simulink model "Assignment_1"  (R2022b)
settings: Solver=FixedStepAuto  StartTime=0.0  StopTime=10.0  FixedStep=1e-3  RelTol=1e-3  EnableMultiTasking=on
settings Model: ExtModeTrigDuration=5  Creator=rebec  LastModifiedBy=rebec
settings OptimizationCC: EnhancedBackFolding=on  PassReuseOutputArgsAs=Individual arguments  ZeroExternalMemoryAtStartup=off  ZeroInternalMemoryAtStartup=off  MaxStackSize=64  OptimizeBlockOrder=speed  DifferentSizesBufferReuse=on  OptimizationCustomize=off  EfficientTunableParamExpr=on
settings DebuggingCC: ParameterTunabilityLossMsg=error
settings HardwareCC: ProdBitPerPointer=32  ProdBitPerSizeT=32  ProdBitPerPtrDiffT=32  ProdLargestAtomicInteger=Long  ProdLargestAtomicFloat=Double  ProdWordSize=32  ProdHWDeviceType=ARM Compatible->ARM Cortex
settings SFSimCC: MATLABDynamicMemAlloc=off
settings RTWCC: Description=Embedded Coder  SystemTargetFile=ert.tlc  HardwareBoard=NXP FRDM-K64F  TLCOptions="-aInlineSetEventsForThisBaseRateFcn=TLC_FALSE -aSuppressMultiTaskScheduler=TLC_FALSE  -aRateBasedStepFcn=0"  TemplateMakefile=ert_default_tmf  Toolchain=GNU Tools for ARM Embedded Processors
settings CodeAppCC: ForceParamTrailComments=on  IgnoreCustomStorageClasses=off  OperatorAnnotations=on  SimulinkDataObjDesc=on  SFDataObjDesc=on  InsertBlockDesc=on
settings ERTTargetCC: ExtModeTransport=4  ExtModeMexFile=sendToCommService

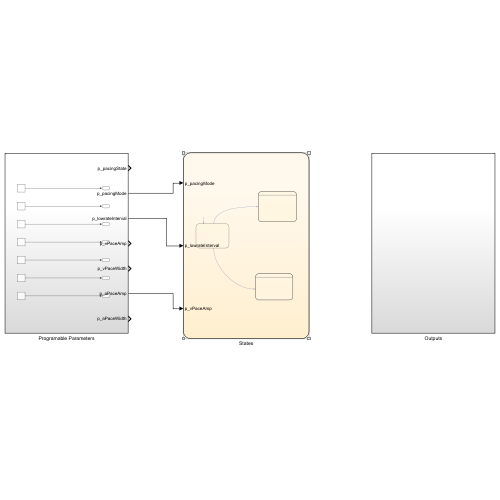
[thumbnail: Simulink's stored preview of the top-level diagram]
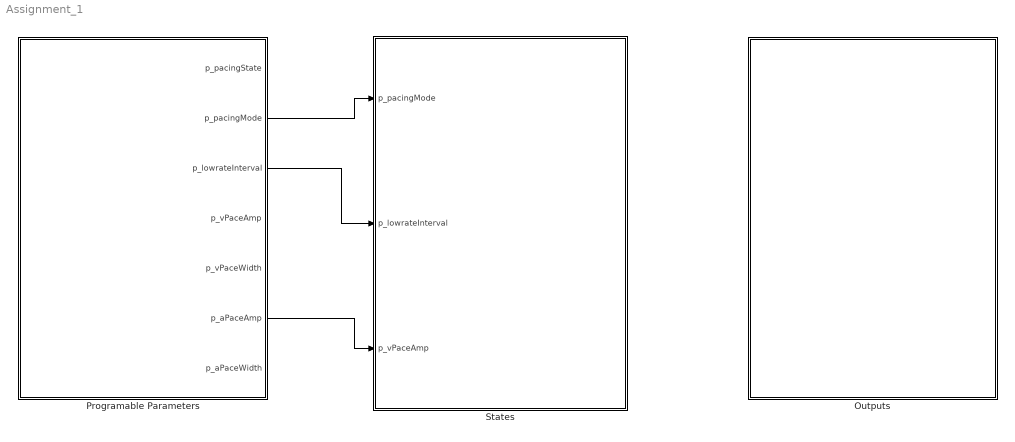
== system Assignment_1 ==
  Outputs : Subsystem
  Programable Parameters : Subsystem
  States : Stateflow chart  TreatAsAtomicUnit=on
  wires:
  Programable Parameters/2(p_pacingMode) -> States/1(p_pacingMode)
  Programable Parameters/6(p_aPaceAmp) -> States/3(p_vPaceAmp)
  Programable Parameters/3(p_lowrateInterval) -> States/2(p_lowrateInterval)

== system Assignment_1/Outputs ==

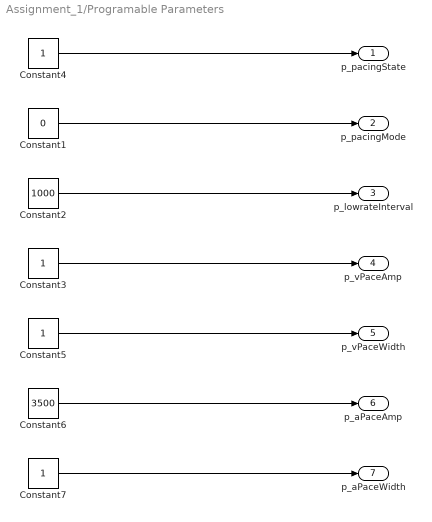
== system Assignment_1/Programable Parameters ==
  Constant1 : Constant  Value=0  OutDataTypeStr=boolean
  Constant2 : Constant  Value=1000
  Constant{3..5,7} (4 alike) : Constant
  Constant6 : Constant  Value=3500
  p_pacingState : Outport
  p_pacingMode : Outport  Port=2
  p_lowrateInterval : Outport  Port=3
  p_vPaceAmp : Outport  Port=4
  p_vPaceWidth : Outport  Port=5
  p_aPaceAmp : Outport  Port=6
  p_aPaceWidth : Outport  Port=7
  wires:
  Constant4/1 -> p_pacingState/1
  Constant3/1 -> p_vPaceAmp/1
  Constant2/1 -> p_lowrateInterval/1
  Constant1/1 -> p_pacingMode/1
  Constant5/1 -> p_vPaceWidth/1
  Constant6/1 -> p_aPaceAmp/1
  Constant7/1 -> p_aPaceWidth/1

== stateflow chart Assignment_1/States ==
  state AOO
    state Pacing
      entry:
      PACE_CHARGE_CTRL = 0;
      PACE_GND_CTRL = 1;
      ATR_PACE_CTRL = 1;
      ATR_GND_CTRL = 0;
      Z_ATR_CTRL = 0;
      Z_VENT_CTRL = 0;
      VENT_GND_CTRL = 0;
      VENT_PACE_CTRL = 0;
    state Charging
      entry:
      ATR_PACE_CTRL = 0;
      VENT_PACE_CTRL = 0;
      PACING_REF_ PWM = ((p_aPaceAmp - 300)/10)/5;
      PACE_CHARGE_CTRL = 1;
    state Discharging
      entry:
      PACE_GND_CTRL = 1;
      VENT_PACE_CTRL = 0;
      Z_ATR_CTRL = 0;
      Z_VENT_CTRL = 0;
      ATR_PACE_CTRL = 0;
      ATR_GND_CTRL = 1;
      VENT_GND_CTRL = 0;
    (default) -> AOO.Charging
    AOO.Charging -> AOO.Pacing : after(p_lowrateInterval, msec)
    AOO.Discharging -> AOO.Charging
    AOO.Pacing -> AOO.Discharging : after(p_lowrateInterval, msec)
  state Start_State
    entry:
    Mode = p_pacingMode;
  state VOO
    state Charging
      entry:
      ATR_PACE_CTRL = 0;
      VENT_PACE_CTRL = 0;
      PACING_REF_ PWM;
      PACE_CHARGE_CTRL = 1;
    state Pacing
      entry:
      PACE_CHARGE_CTRL = 0;
      PACE_GND_CTRL = 1;
      ATR_PACE_CTRL = 0;
      ATR_GND_CTRL = 0;
      Z_ATR_CTRL = 0;
      Z_VENT_CTRL = 0;
      VENT_GND_CTRL = 0;
      VENT_PACE_CTRL = 1;
    state Discharging
      entry:
      PACE_GND_CTRL = 1;
      VENT_PACE_CTRL = 0;
      Z_ATR_CTRL = 0;
      Z_VENT_CTRL = 0;
      ATR_PACE_CTRL = 0;
      ATR_GND_CTRL = 0;
      VENT_GND_CTRL = 1;
    (default) -> VOO.Charging
    VOO.Charging -> VOO.Pacing
    VOO.Discharging -> VOO.Charging
    VOO.Pacing -> VOO.Discharging
  Start_State -> AOO [order 1]
  (default) -> Start_State
  Start_State -> VOO [order 2]
  data: p_pacingMode input; p_lowrateInterval input; p_vPaceAmp input
